simulink model "Solar_Cell_Model"  (R2021b)
settings: Solver=VariableStepAuto  StartTime=0.0  StopTime=0.6  RelTol=1e-3
libraries: simulink x1
settings Model: Creator=ftmmim  LastModifiedBy=ftmmim

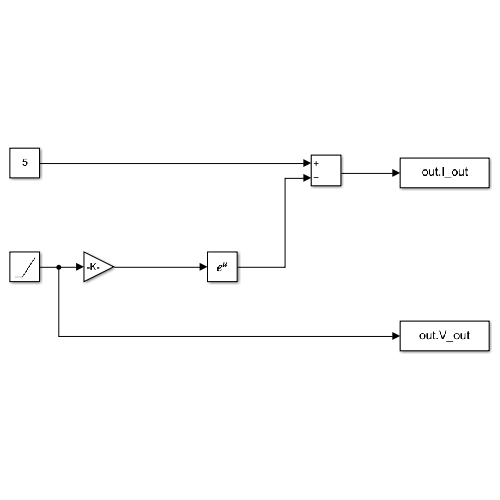
[thumbnail: Simulink's stored preview of the top-level diagram]
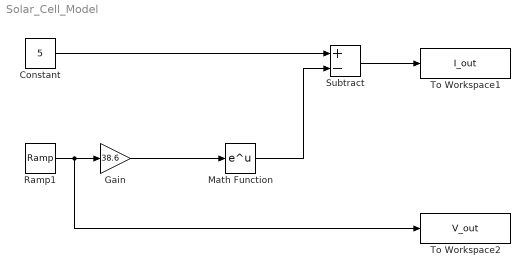
== system Solar_Cell_Model ==
  Constant : Constant  Value=5
  Gain : Gain  Gain=38.6
  Math Function : Math  SaturateOnIntegerOverflow=on
  Ramp1 : simulink/Sources/Ramp  slope=1  start=0  InitialOutput=0
  Subtract : Sum  Inputs=+-
  To Workspace1 : ToWorkspace  VariableName=I_out  SampleTime=-1
  To Workspace2 : ToWorkspace  VariableName=V_out  SampleTime=-1
  wires:
  Ramp1/1 -> To Workspace2/1, Gain/1
  Gain/1 -> Math Function/1
  Math Function/1 -> Subtract/2
  Constant/1 -> Subtract/1
  Subtract/1 -> To Workspace1/1
